simulink model "batch_events_3_super_1_sm_master"  (R2021b)
settings: Solver=ode4  StartTime=0.0  StopTime=inf  FixedStep=0.001  RelTol=1e-3  EnableMultiTasking=on
model workspace (MATLAB code in the model file):
  | % Add the class folders into the path.
  | addpath src/model
  | addpath src/utils
  | 
  | %% Loading data from files.
  | % Data for supervisor 1.
  | utils1 = StateMachineUtils;
  | 
  | % From TCT: Load all events' number.
  | utils1 = utils1.loadEventsInAds('resources/tct/ALLEVENT.ADS');
  | 
  | % From TCT: Disabled events in each state.
  | utils1 = utils1.loadDisabledEventsInPdt('resources/tct/supervisor1/DATA_SIMSUP1_MG1.PDT');
  | 
  | % From TCT: Transition matrix.
  | utils1 = utils1.loadTransitionsInAds('resources/tct/supervisor1/SIMSUP1_MG1.ADS');
  | 
  | % Parameters for the block.
  | encodedStates1 = StateEncoder.encode(utils1.statesArray);
  | 
  | transitions1 = utils1.transitions;
  | 
  | allEvents1 = utils1.eventsArray;
  | 
  | % Data for supervisor 2.
  | utils2 = StateMachineUtils;
  | 
  | % From TCT: Load all events' number.
  | utils2 = utils2.loadEventsInAds('resources/tct/ALLEVENT.ADS');
  | 
  | % From TCT: Disabled events in each state.
  | utils2 = utils2.loadDisabledEventsInPdt('resources/tct/supervisor2/DATA_SIMSUP2_MG1.PDT');
  | 
  | % From TCT: Transition matrix.
  | utils2 = utils2.loadTransitionsInAds('resources/tct/supervisor2/SIMSUP2_MG1.ADS');
  | 
  | % Parameters for the block.
  | encodedStates2 = StateEncoder.encode(utils2.statesArray);
  | 
  | transitions2 = utils2.transitions;
  | 
  | allEvents2 = utils2.eventsArray;
  | 
  | % Data for supervisor 3.
  | utils3 = StateMachineUtils;
  | 
  | % From TCT: Load all events' number.
  | utils3 = utils3.loadEventsInAds('resources/tct/ALLEVENT.ADS');
  | 
  | % From TCT: Disabled events in each state.
  | utils3 = utils3.loadDisabledEventsInPdt('resources/tct/supervisor3/DATA_SIMSUP3_MG1.PDT');
  | 
  | % From TCT: Transition matrix.
  | utils3 = utils3.loadTransitionsInAds('resources/tct/supervisor3/SIMSUP3_MG1.ADS');
  | 
  | % Parameters for the block.
  | encodedStates3 = StateEncoder.encode(utils3.statesArray);
  | 
  | transitions3 = utils3.transitions;
  | 
  | allEvents3 = utils3.eventsArray;
libraries: opal_lib x3
Description:
  | Model of a simple control system for use iin training.
settings Model: Creator=Paul Baracos  LastModifiedBy=andrerangel
settings SolverCC: AlgebraicLoopSolver=TrustRegion
settings DataIOCC: LimitDataPoints=on  SaveFormat=Array  SignalLoggingSaveFormat=ModelDataLogs  SaveOutput=off  SaveTime=off  ReturnWorkspaceOutputs=off  SignalLoggingName=sigsOut
settings OptimizationCC: BlockReduction=off  BooleanDataType=off  OptimizeBlockIOStorage=off  BufferReuse=off  ExpressionFolding=off  LocalBlockOutputs=off  InitFltsAndDblsToZero=on  LifeSpan=inf
settings DebuggingCC: SaveWithParameterizedLinksMsg=none  UnderspecifiedInitializationDetection=Classic  MergeDetectMultiDrivingBlocksExec=none  SignalResolutionControl=TryResolveAllWithWarning  MultiTaskDSMMsg=warning  MultiTaskCondExecSysMsg=none  FcnCallInpInsideContextMsg=warning  SFUnexpectedBacktrackingDiag=warning  SFNoUnconditionalDefaultTransitionDiag=warning  SFExecutionAtInitializationDiag=none  SFMachineParentedDataDiag=warning  ArithmeticOperatorsInVariantConditions=warning
settings HardwareCC: ProdBitPerPointer=32  ProdBitPerSizeT=32  ProdBitPerPtrDiffT=32  ProdLargestAtomicFloat=None  ProdIntDivRoundTo=Undefined  ProdEndianess=Unspecified  ProdWordSize=32  ProdHWDeviceType=32-bit Generic  TargetUnknown=on
settings ModelReferenceCC: PropagateSignalLabelsOutOfModel=off
settings SFSimCC: SimUseLocalCustomCode=off  CustomCodeUndefinedFunction=UseInterfaceOnly
settings RTWCC: GenCodeOnly=on  RTWUseLocalCustomCode=off
settings CodeAppCC: StateflowObjectComments=on
settings GRTTargetCC: TargetFcnLib=ansi_tfl_tmw.mat  TargetLangStandard=C89/C90 (ANSI)  CombineOutputUpdateFcns=off  GRTInterface=on
settings ConfigComp: CovMetricSettings=dw  CovSaveCumulativeToWorkspaceVar=on  CovSaveSingleToWorkspaceVar=on  CovExternalEMLEnable=off

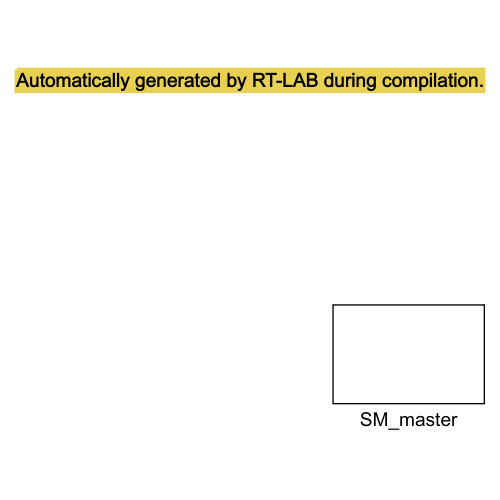
[thumbnail: Simulink's stored preview of the top-level diagram]
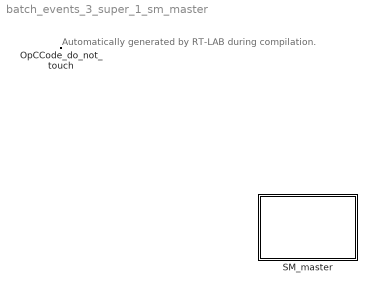
== system batch_events_3_super_1_sm_master ==
  note: Automatically generated by RT-LAB during compilation.
  OpCCode_do_not_touch : opal_lib/Communication/OpCCode  SystemSampleTime=-1  VariantActivationTime=update diagram  Latency=0  AutoFrameSizeCalculation=off
  SM_master : Subsystem

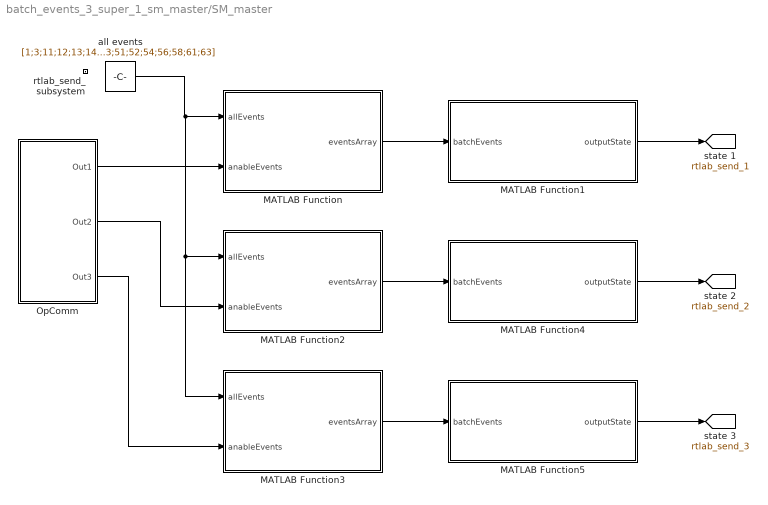
== system batch_events_3_super_1_sm_master/SM_master ==
  MATLAB Function : MATLAB Function  TreatAsAtomicUnit=on
  MATLAB Function1 : MATLAB Function  TreatAsAtomicUnit=on
  MATLAB Function2 : MATLAB Function  TreatAsAtomicUnit=on
  MATLAB Function3 : MATLAB Function  TreatAsAtomicUnit=on
  MATLAB Function4 : MATLAB Function  TreatAsAtomicUnit=on
  MATLAB Function5 : MATLAB Function  TreatAsAtomicUnit=on
  OpComm : Subsystem
      mask init:
      | opmaskdisplay('maskdisplay_block',gcb,'disp(''OpComm'')');
      mask Display:
      | patch([0 0.5 0.7 0],[1 1 0 0],[0.7 0.75 0.9]);
      | patch([1 0.53 0.73 1],[1 1 0 0],[1 0.8 0.7]);
      | plot([0 0 1 1 0],[0 1 1 0 0]);
      | disp('OpComm')
  all events : Constant  Value=[1;3;11;12;13;14;16;21;23;25;27;31;32;33;34;36;41;43;51;52;54;56;58;61;63]
  rtlab_send_subsystem : Subsystem  Priority=-100
      mask Display: text(0,0,'');
  tag scope: rtlab_send_1=global, rtlab_send_2=global, rtlab_send_3=global
  wires:
  OpComm/1(Out1) -> MATLAB Function/2(anableEvents)
  MATLAB Function/1(eventsArray) -> MATLAB Function1/1(batchEvents)
  MATLAB Function1/1(outputState) -> [rtlab_send_1]
  all events/1 -> MATLAB Function3/1(allEvents), MATLAB Function2/1(allEvents), MATLAB Function/1(allEvents)
  OpComm/2(Out2) -> MATLAB Function2/2(anableEvents)
  OpComm/3(Out3) -> MATLAB Function3/2(anableEvents)
  MATLAB Function2/1(eventsArray) -> MATLAB Function4/1(batchEvents)
  MATLAB Function3/1(eventsArray) -> MATLAB Function5/1(batchEvents)
  MATLAB Function5/1(outputState) -> [rtlab_send_3]
  MATLAB Function4/1(outputState) -> [rtlab_send_2]

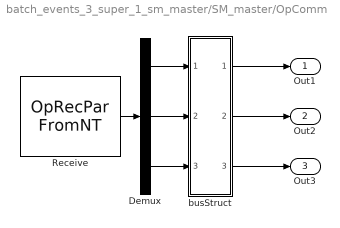
== system batch_events_3_super_1_sm_master/SM_master/OpComm ==
  Demux : Demux  Outputs="[3  3  3]"
  Receive : opal_lib/Communication/OpRecPar FromNT  Data_width=9  InitialConditions=[14;23;36;14;32;36;14;32;36]
  busStruct : Subsystem
  Out1 : Outport
  Out2 : Outport  Port=2
  Out3 : Outport  Port=3
  wires:
  Demux/3 -> busStruct/3(In3)
  Demux/2 -> busStruct/2(In2)
  Demux/1 -> busStruct/1(In1)
  busStruct/3(Out3) -> Out3/1
  busStruct/2(Out2) -> Out2/1
  busStruct/1(Out1) -> Out1/1
  Receive/1 -> Demux/1

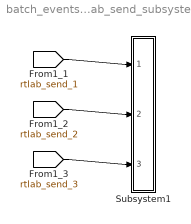
== system batch_events_3_super_1_sm_master/SM_master/rtlab_send_subsystem ==
  Subsystem1 : Subsystem
  wires:
  [rtlab_send_1] -> Subsystem1/1(In1)
  [rtlab_send_2] -> Subsystem1/2(In2)
  [rtlab_send_3] -> Subsystem1/3(In3)

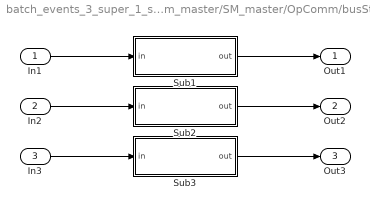
== system batch_events_3_super_1_sm_master/SM_master/OpComm/busStruct ==
  In1 : Inport
  In2 : Inport  Port=2
  In3 : Inport  Port=3
  Sub1 : Subsystem
  Sub2 : Subsystem
  Sub3 : Subsystem
  Out1 : Outport
  Out2 : Outport  Port=2
  Out3 : Outport  Port=3
  wires:
  Sub3/1(out) -> Out3/1
  In3/1 -> Sub3/1(in)
  Sub2/1(out) -> Out2/1
  In2/1 -> Sub2/1(in)
  Sub1/1(out) -> Out1/1
  In1/1 -> Sub1/1(in)

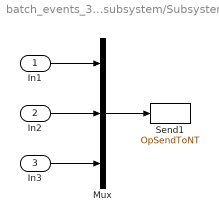
== system batch_events_3_super_1_sm_master/SM_master/rtlab_send_subsystem/Subsystem1 ==
  In1 : Inport
  In2 : Inport  Port=2
  In3 : Inport  Port=3
  Mux : Mux  Inputs=3
  Send1 : opal_lib/Communication/OpSendToNT  Acqu_group=1
  wires:
  Mux/1 -> Send1/1
  In1/1 -> Mux/1
  In2/1 -> Mux/2
  In3/1 -> Mux/3

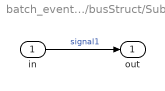
== system batch_events_3_super_1_sm_master/SM_master/OpComm/busStruct/Sub1 ==
  in : Inport
  out : Outport
  wires:
  in/1 -> out/1  "signal1"

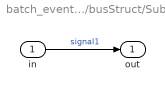
== system batch_events_3_super_1_sm_master/SM_master/OpComm/busStruct/Sub2 ==
  in : Inport
  out : Outport
  wires:
  in/1 -> out/1  "signal1"

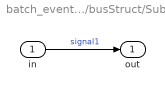
== system batch_events_3_super_1_sm_master/SM_master/OpComm/busStruct/Sub3 ==
  in : Inport
  out : Outport
  wires:
  in/1 -> out/1  "signal1"

== matlab function batch_events_3_super_1_sm_master/SM_master/MATLAB Function1 ==
  data: batchEvents input; outputState output; encodedStates1 parameter; transitions1 parameter; allEvents1 parameter
function outputState  = stateMachine1(batchEvents, encodedStates1, transitions1, allEvents1)
% State Machine with parameters from files.
% Receives a batch of events and process one event at time, starting with
% the event of index 1.
% batchEvents: array with 0s and 1s where 1 is the enabled event while 0,
% is disabled event;
% allEvents: numbers of the events;
% transitions: matrix of transitions;
% encodedStates: Encoded states array to be decoded before the pass it to
% StateMachines as an argument.

% Initialize a persistent object. Its value will not be erased as this
% block finishes.
persistent stateMachine

% Assign the persistent object to the StateMachine class with data passed
% as parameters.
if (isempty(stateMachine))
    statesArray = StateEncoder.decode(encodedStates1);                        
    stateMachine = StateMachine(statesArray, transitions1, allEvents1);
end

anabledEvents = allEvents1(logical(batchEvents));

% loop through an array of events:
for i=1:length(anabledEvents)
    stateMachine.inputEvent = anabledEvents(i);
end
outputState = double(stateMachine.currentState.number);

== matlab function batch_events_3_super_1_sm_master/SM_master/MATLAB Function ==
  data: allEvents input; eventsArray output; anableEvents input
function eventsArray = eventsGenerator(allEvents, anableEvents)

[~, indexes] = ismember(anableEvents, allEvents);

eventsArray = zeros(length(allEvents), 1);

eventsArray(indexes) = 1;

== matlab function batch_events_3_super_1_sm_master/SM_master/MATLAB Function2 ==
  data: allEvents input; eventsArray output; anableEvents input
function eventsArray = eventsGenerator(allEvents, anableEvents)

[~, indexes] = ismember(anableEvents, allEvents);

eventsArray = zeros(length(allEvents), 1);

eventsArray(indexes) = 1;

== matlab function batch_events_3_super_1_sm_master/SM_master/MATLAB Function3 ==
  data: allEvents input; eventsArray output; anableEvents input
function eventsArray = eventsGenerator(allEvents, anableEvents)

[~, indexes] = ismember(anableEvents, allEvents);

eventsArray = zeros(length(allEvents), 1);

eventsArray(indexes) = 1;

== matlab function batch_events_3_super_1_sm_master/SM_master/MATLAB Function4 ==
  data: batchEvents input; outputState output; encodedStates2 parameter; transitions2 parameter; allEvents2 parameter
function outputState  = stateMachine2(batchEvents, encodedStates2, transitions2, allEvents2)
% State Machine with parameters from files.
% Receives a batch of events and process one event at time, starting with
% the event of index 1.
% batchEvents: array with 0s and 1s where 1 is the enabled event while 0,
% is disabled event;
% allEvents: numbers of the events;
% transitions: matrix of transitions;
% encodedStates: Encoded states array to be decoded before the pass it to
% StateMachines as an argument.

% Initialize a persistent object. Its value will not be erased as this
% block finishes.
persistent stateMachine

% Assign the persistent object to the StateMachine class with data passed
% as parameters.
if (isempty(stateMachine))
    statesArray = StateEncoder.decode(encodedStates2);                        
    stateMachine = StateMachine(statesArray, transitions2, allEvents2);
end

anabledEvents = allEvents2(logical(batchEvents));

% loop through an array of events:
for i=1:length(anabledEvents)
    stateMachine.inputEvent = anabledEvents(i);
end
outputState = double(stateMachine.currentState.number);

== matlab function batch_events_3_super_1_sm_master/SM_master/MATLAB Function5 ==
  data: batchEvents input; outputState output; encodedStates3 parameter; transitions3 parameter; allEvents3 parameter
function outputState  = stateMachine3(batchEvents, encodedStates3, transitions3, allEvents3)
% State Machine with parameters from files.
% Receives a batch of events and process one event at time, starting with
% the event of index 1.
% batchEvents: array with 0s and 1s where 1 is the enabled event while 0,
% is disabled event;
% allEvents: numbers of the events;
% transitions: matrix of transitions;
% encodedStates: Encoded states array to be decoded before the pass it to
% StateMachines as an argument.

% Initialize a persistent object. Its value will not be erased as this
% block finishes.
persistent stateMachine

% Assign the persistent object to the StateMachine class with data passed
% as parameters.
if (isempty(stateMachine))
    statesArray = StateEncoder.decode(encodedStates3);                        
    stateMachine = StateMachine(statesArray, transitions3, allEvents3);
end

anabledEvents = allEvents3(logical(batchEvents));

% loop through an array of events:
for i=1:length(anabledEvents)
    stateMachine.inputEvent = anabledEvents(i);
end
outputState = double(stateMachine.currentState.number);
